simulink model "SimulacionesV2016"  (Simulink 8.8)
settings: Solver=VariableStepAuto  StartTime=1  StopTime=TiempoSim  FixedStep=1/(FrecRuido*100)  RelTol=1e-3
values from neighbouring files (symbols this model uses):
  FrecRuidoBloque = 2*FrecRuido    (= 31.8309886184)    [Simulaciones.m]
  Fs = 3*FrecRuidoBloque    (= 95.4929658551)    [Simulaciones.m]
  Is = 1e3    (= 1000)    [Simulaciones.m]
  K = Is*wn^2    (= 0.1)    [Simulaciones.m]
  Kd = 2*psi*wn*Is    (= 14)    [Simulaciones.m]
  wc = wn*100    (= 1)    [Simulaciones.m]
libraries: simulink x3
settings Model: SuppressorTable=22 serialization::archive 11 0 3 0 0 0 11 0  Creator=root  LastModifiedBy=root
settings DataIOCC: LimitDataPoints=off  SaveFormat=Dataset  SignalLoggingSaveFormat=Dataset
settings OptimizationCC: LifeSpan=auto
settings DebuggingCC: UnderspecifiedInitializationDetection=Simplified  MergeDetectMultiDrivingBlocksExec=error  FcnCallInpInsideContextMsg=error  StateNameClashWarn=none  SFUnexpectedBacktrackingDiag=error  SFNoUnconditionalDefaultTransitionDiag=error  SFExecutionAtInitializationDiag=warning
settings HardwareCC: ProdBitPerLong=64  ProdBitPerPointer=64  ProdBitPerSizeT=64  ProdBitPerPtrDiffT=64  ProdLargestAtomicFloat=Float  ProdIntDivRoundTo=Zero  ProdEndianess=LittleEndian  ProdWordSize=64  ProdHWDeviceType=Intel->x86-64 (Linux 64)
settings ModelReferenceCC: PropagateSignalLabelsOutOfModel=on
settings GRTTargetCC: TargetLangStandard=C99 (ISO)  GeneratePreprocessorConditionals=Use local settings  CombineOutputUpdateFcns=on  GRTInterface=off
settings ConfigComp: CovMetricSettings=dwe  CovHtmlReporting=off  CovSaveCumulativeToWorkspaceVar=off  CovSaveSingleToWorkspaceVar=off  CovExternalEMLEnable=on

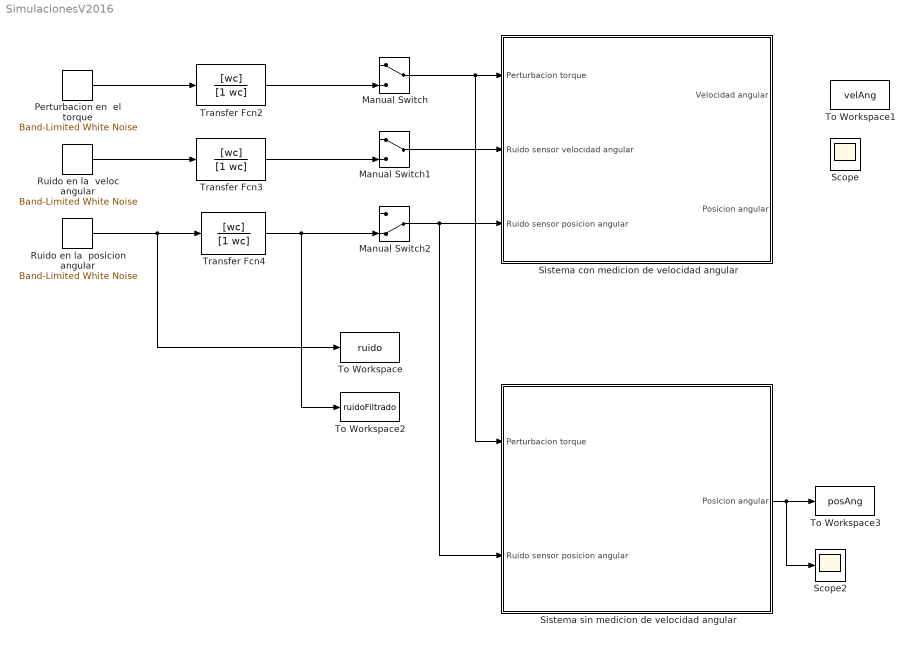
== system SimulacionesV2016 ==
  Manual Switch : ManualSwitch
  Manual Switch1 : ManualSwitch
  Manual Switch2 : ManualSwitch  CurrentSetting=0
  Perturbacion en  el torque : simulink/Sources/Band-Limited White Noise  Cov=A  Ts=1/FrecRuidoBloque  seed=[10000]
  Ruido en la  posicion angular : simulink/Sources/Band-Limited White Noise  Cov=A  Ts=1/FrecRuidoBloque  seed=[50000]
  Ruido en la  veloc angular : simulink/Sources/Band-Limited White Noise  Cov=A  Ts=1/FrecRuidoBloque  seed=[23341]
  Scope : Scope
  Scope2 : Scope
  Sistema con medicion de velocidad angular : Subsystem
  Sistema sin medicion de velocidad angular : Subsystem
  To Workspace : ToWorkspace  VariableName=ruido  SampleTime=1/Fs
  To Workspace1 : ToWorkspace  VariableName=velAng  SampleTime=1/Fs
      settings: Save2DSignal=2-D array (concatenate along first dimension)
  To Workspace2 : ToWorkspace  VariableName=ruidoFiltrado  SampleTime=1/Fs
  To Workspace3 : ToWorkspace  VariableName=posAng  SampleTime=1/Fs
      settings: Save2DSignal=2-D array (concatenate along first dimension)
  Transfer Fcn2 : TransferFcn  Numerator=[wc]  Denominator=[1 wc]
  Transfer Fcn3 : TransferFcn  Numerator=[wc]  Denominator=[1 wc]
  Transfer Fcn4 : TransferFcn  Numerator=[wc]  Denominator=[1 wc]
  wires:
  Transfer Fcn2/1 -> Manual Switch/2
  Transfer Fcn3/1 -> Manual Switch1/2
  Ruido en la  veloc angular/1 -> Transfer Fcn3/1
  Ruido en la  posicion angular/1 -> To Workspace/1, Transfer Fcn4/1
  Manual Switch/1 -> Sistema sin medicion de velocidad angular/1(Perturbacion torque), Sistema con medicion de velocidad angular/1(Perturbacion torque)
  Manual Switch1/1 -> Sistema con medicion de velocidad angular/2(Ruido sensor velocidad angular)
  Perturbacion en  el torque/1 -> Transfer Fcn2/1
  Transfer Fcn4/1 -> To Workspace2/1, Manual Switch2/2
  Manual Switch2/1 -> Sistema sin medicion de velocidad angular/2(Ruido sensor posicion angular), Sistema con medicion de velocidad angular/3(Ruido sensor posicion angular)
  Sistema sin medicion de velocidad angular/1(Posicion angular) -> Scope2/1, To Workspace3/1

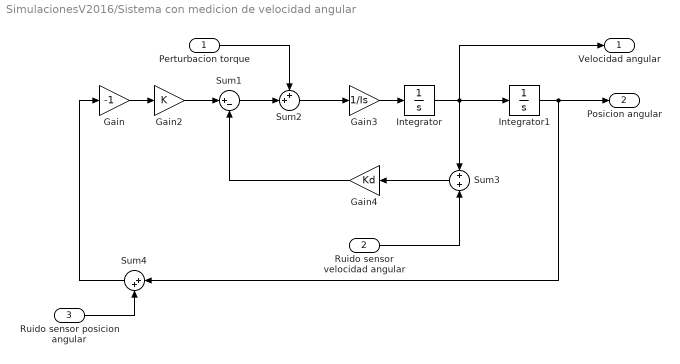
== system SimulacionesV2016/Sistema con medicion de velocidad angular ==
  Perturbacion torque : Inport
  Ruido sensor velocidad angular : Inport  Port=2
  Ruido sensor posicion angular : Inport  Port=3
  Gain : Gain  Gain=-1
  Gain2 : Gain  Gain=K
  Gain3 : Gain  Gain=1/Is
  Gain4 : Gain  Gain=Kd
  Integrator : Integrator
  Integrator1 : Integrator
  Sum1 : Sum  Inputs=|+-
  Sum2 : Sum  Inputs=++|
  Sum3 : Sum  Inputs=+|+
  Sum4 : Sum  Inputs=|++
  Velocidad angular : Outport
  Posicion angular : Outport  Port=2
  wires:
  Sum4/1 -> Gain/1
  Ruido sensor posicion angular/1 -> Sum4/2
  Gain/1 -> Gain2/1
  Perturbacion torque/1 -> Sum2/1
  Ruido sensor velocidad angular/1 -> Sum3/2
  Gain3/1 -> Integrator/1
  Sum3/1 -> Gain4/1
  Integrator1/1 -> Posicion angular/1, Sum4/1
  Gain2/1 -> Sum1/1
  Sum1/1 -> Sum2/2
  Sum2/1 -> Gain3/1
  Gain4/1 -> Sum1/2
  Integrator/1 -> Velocidad angular/1, Sum3/1, Integrator1/1

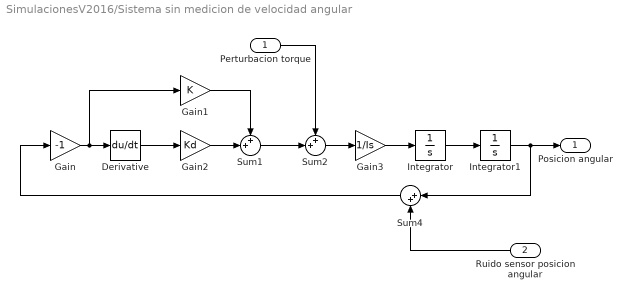
== system SimulacionesV2016/Sistema sin medicion de velocidad angular ==
  Perturbacion torque : Inport
  Ruido sensor posicion angular : Inport  Port=2
  Derivative : Derivative
  Gain : Gain  Gain=-1
  Gain1 : Gain  Gain=K
  Gain2 : Gain  Gain=Kd
  Gain3 : Gain  Gain=1/Is
  Integrator : Integrator
  Integrator1 : Integrator
  Sum1 : Sum  Inputs=++|
  Sum2 : Sum  Inputs=++|
  Sum4 : Sum  Inputs=|++
  Posicion angular : Outport
  wires:
  Sum4/1 -> Gain/1
  Perturbacion torque/1 -> Sum2/1
  Gain3/1 -> Integrator/1
  Integrator/1 -> Integrator1/1
  Integrator1/1 -> Posicion angular/1, Sum4/1
  Sum2/1 -> Gain3/1
  Sum1/1 -> Sum2/2
  Gain/1 -> Gain1/1, Derivative/1
  Derivative/1 -> Gain2/1
  Gain1/1 -> Sum1/1
  Gain2/1 -> Sum1/2
  Ruido sensor posicion angular/1 -> Sum4/2
